simulink model "PreScan_Vissim_Python_0_cs_old"  (R2017b)
settings: Solver=ode5  StartTime=0.0  StopTime=inf  FixedStep=1/200  RelTol=1e-3
PreLoadFcn:
  | mbxruntime.callbacks.PreLoadFcn(bdroot);
PostLoadFcn:
  | mbxruntime.callbacks.PostLoadFcn(bdroot);
InitFcn:
  | mbxruntime.callbacks.InitFcn(bdroot);
StartFcn:
  | mbxruntime.callbacks.StartFcn(bdroot);
StopFcn:
  | mbxruntime.callbacks.StopFcn(bdroot);
model workspace (MAT data in the model file):
  mbox_table : struct (value not decoded)
  model_closed = 0
  sim_status = 0
undefined symbols (not defined in the file or in its folder): DiscIntNeverNeededParam
libraries: simulink x37, simulink_extras x12, PreScanSimulinkLibrary x11, dspnetwork x2, etargetslib x1, simulink_need_slupdate x1
(part 6 of 6)

== system PreScan_Vissim_Python_0_cs_old/Toyota_Yaris_Hatchback_1/Trajectories/Traj2State1/Traj2State2/Traj2MuxState_Ext/demux ==
  traj : Inport
  Demux : Demux  Outputs=18
  x : Outport
  y : Outport  Port=2
  z : Outport  Port=3
  velx : Outport  Port=4
  vely : Outport  Port=5
  velz : Outport  Port=6
  R : Outport  Port=7
  P : Outport  Port=8
  Y : Outport  Port=9
  velR : Outport  Port=10
  velP : Outport  Port=11
  velY : Outport  Port=12
  accx : Outport  Port=13
  accy : Outport  Port=14
  accz : Outport  Port=15
  accR : Outport  Port=16
  accP : Outport  Port=17
  accY : Outport  Port=18
  wires:
  Demux/18 -> accY/1
  Demux/17 -> accP/1
  Demux/16 -> accR/1
  Demux/15 -> accz/1
  Demux/14 -> accy/1
  Demux/13 -> accx/1
  Demux/12 -> velY/1
  Demux/11 -> velP/1
  Demux/10 -> velR/1
  Demux/9 -> velz/1
  Demux/8 -> vely/1
  Demux/7 -> velx/1
  Demux/6 -> Y/1
  Demux/5 -> P/1
  traj/1 -> Demux/1
  Demux/4 -> R/1
  Demux/3 -> z/1
  Demux/2 -> y/1
  Demux/1 -> x/1

== system PreScan_Vissim_Python_0_cs_old/Fiat_Bravo_Hatchback_1/Dynamics_Simple/Chassis/Bicycle_model_[XYZ]/X_Motion/Max RPM and zero- velocity detection/Configurable Subsystem ==
  Step : Step  Time=0.0001  Before=1  After=0  SampleTime=0
  Out1 : Outport
  wires:
  Step/1 -> Out1/1

== system PreScan_Vissim_Python_0_cs_old/Fiat_Bravo_Hatchback_1/Dynamics_Simple/Chassis/Bicycle_model_[XYZ]/X_Motion/Max RPM and zero- velocity detection/SR-Memory ==
  Signal : Inport
  Set : Inport  Port=2
  Reset : Inport  Port=3
  Constant : Constant  Value=0
  Detect Rise Positive : simulink/Logic and Bit Operations/Detect Rise Positive  vinit=0  InputProcessing=Inherited  OutDataTypeStr=uint8
  Detect Rise Positive1 : simulink/Logic and Bit Operations/Detect Rise Positive  vinit=0  InputProcessing=Inherited  OutDataTypeStr=uint8
  Manual Switch : ManualSwitch
  Manual Switch1 : ManualSwitch
  Switch : Switch  Criteria=u2 ~= 0
  Switch1 : Switch  Criteria=u2 ~= 0
  Unit Delay : UnitDelay  SampleTime=-1
  Out : Outport
  wires:
  Constant/1 -> Switch1/1
  Switch/1 -> Switch1/3
  Switch1/1 -> Unit Delay/1, Out/1
  Manual Switch1/1 -> Switch1/2
  Reset/1 -> Manual Switch1/2, Detect Rise Positive1/1
  Detect Rise Positive1/1 -> Manual Switch1/1
  Signal/1 -> Switch/1
  Unit Delay/1 -> Switch/3
  Set/1 -> Detect Rise Positive/1, Manual Switch/2
  Detect Rise Positive/1 -> Manual Switch/1
  Manual Switch/1 -> Switch/2

== system PreScan_Vissim_Python_0_cs_old/Toyota_Yaris_Hatchback_1/Dynamics_Simple/Chassis/Bicycle_model_[XYZ]/X_Motion/Max RPM and zero- velocity detection/Configurable Subsystem ==
  Step : Step  Time=0.0001  Before=1  After=0  SampleTime=0
  Out1 : Outport
  wires:
  Step/1 -> Out1/1

== system PreScan_Vissim_Python_0_cs_old/Toyota_Yaris_Hatchback_1/Dynamics_Simple/Chassis/Bicycle_model_[XYZ]/X_Motion/Max RPM and zero- velocity detection/SR-Memory ==
  Signal : Inport
  Set : Inport  Port=2
  Reset : Inport  Port=3
  Constant : Constant  Value=0
  Detect Rise Positive : simulink/Logic and Bit Operations/Detect Rise Positive  vinit=0  OutDataTypeStr=uint8
  Detect Rise Positive1 : simulink/Logic and Bit Operations/Detect Rise Positive  vinit=0  OutDataTypeStr=uint8
  Manual Switch : ManualSwitch
  Manual Switch1 : ManualSwitch
  Switch : Switch  Criteria=u2 ~= 0
  Switch1 : Switch  Criteria=u2 ~= 0
  Unit Delay : UnitDelay  SampleTime=-1
  Out : Outport
  wires:
  Constant/1 -> Switch1/1
  Switch/1 -> Switch1/3
  Switch1/1 -> Unit Delay/1, Out/1
  Manual Switch1/1 -> Switch1/2
  Reset/1 -> Manual Switch1/2, Detect Rise Positive1/1
  Detect Rise Positive1/1 -> Manual Switch1/1
  Signal/1 -> Switch/1
  Unit Delay/1 -> Switch/3
  Set/1 -> Detect Rise Positive/1, Manual Switch/2
  Detect Rise Positive/1 -> Manual Switch/1
  Manual Switch/1 -> Switch/2

== matlab function PreScan_Vissim_Python_0_cs_old/Toyota_Yaris_Hatchback_1/MATLAB Function6 ==
  data: u input; y1 output; y2 output; y3 output; y4 output; y5 output
function [y1,y2,y3,y4,y5]= fcn(u)

y1 = u(1);
y2 = u(2);
y3 = u(3);
y4 = u(4);
y5 = u(5);

== matlab function PreScan_Vissim_Python_0_cs_old/Toyota_Yaris_Hatchback_1/MATLAB Function1 ==
  data: x input; y output
function y = fcn(x)
y=0;
if (x>=750)
    y = 1;
end

== matlab function PreScan_Vissim_Python_0_cs_old/Toyota_Yaris_Hatchback_1/MATLAB Function ==
  data: u input; y output
function y = fcn(u)

y = u(1);
%pause(1);

== matlab function PreScan_Vissim_Python_0_cs_old/Toyota_Yaris_Hatchback_1/MATLAB Function7 ==
  data: IDs input; range input; azimuth input; send_data output; vel input; state input; if_collide input; Collid_1 input; Collid_2 input; if_road_end input
function send_data = fcn(IDs,range,azimuth ,vel ,state, if_collide,Collid_1,Collid_2,if_road_end)
coder.extrinsic('mat2str','disp','num2str','bdroot','get_param');


Number_data=10;
pt = 10;


t = num2str(round(get_param(bdroot,'SimulationTime'),pt),['%0' num2str(pt) '.2f ']);
% t = num2str(2.2,['%0.' num2str(pt) 'f ']);

To_add=['{"Time":"' t '", '];


for i=1:Number_data
    Id_name=num2str(i,['%0' num2str(3) '.f ']);
    Id_Colide=num2str(IDs(i),['%0' num2str(pt) '.f ']);
    Ra_Colide=num2str(range(i),['%0' num2str(pt) '.2f ']);
    az_Colide=num2str(azimuth(i),['%0' num2str(pt) '.2f ']);
    Ve_Colide=num2str(vel(i),['%0' num2str(pt) '.2f ']);
    
    
    To_add=[To_add '"Id' Id_name '":"' Id_Colide '", ' ...
                   '"Range' Id_name '":"' Ra_Colide '", ' ...
                   '"Azimuth' Id_name '":"' az_Colide '",' ...
                   '"Velocity' Id_name '":"' Ve_Colide '" '] ;
   if i<Number_data
       To_add=[To_add ', '];
   end
end

To_add=[To_add ', '];

pInput = 15;
pt = 10;
% % % % % % % % % % % % % % % % % 
p = pInput + 7;
state(isnan(state)) = 0;
u = zeros(9,p);
m = num2str([state(:);-1], ['% .' num2str(pInput) 'e ']);
sss = 1:p;
u(1,sss) = m(1,sss);    
u(2,sss) = m(2,sss);
u(3,sss) = m(3,sss);
u(4,sss) = m(4,sss);
u(5,sss) = m(5,sss);





To_add=[To_add '"Position":{"x":' u(1,:) ',"y":' u(2,:) '},' ...
        '"Velocity":' u(3,:) ',' ...
        '"Heading":' u(4,:) ',' ...
        '"Yaw":' u(5,:) ',' ];

% To_add=[To_add '"Position":{"x":' u(1,:) ',"y":' u(2,:) '},' ...
%         '"Velocity":' u(3,:) ',' ...
%         '"Heading":' u(3,:) ',' ...
%         '"Reward":' u(4,:) '}' ];
    
    
if_collide_s=num2str((if_collide),['%0' num2str(pt) '.f ']);
Collid_1_s=num2str(Collid_1,['%0' num2str(pt) '.f ']);
Collid_2_s=num2str(Collid_2,['%0' num2str(pt) '.f ']);

if_road_end_s=num2str((if_road_end),['%0' num2str(pt) '.f ']);


To_add=[To_add '"if_road_end":"' if_road_end_s '",'  ...
                '"if_collide":"' if_collide_s '",'  ...
                '"Collid_1":"' Collid_1_s '",'  ...
                '"Collid_2":"' Collid_2_s '"}'];


len=1306;
send_data = uint8(40*ones(len,1));

send_data = uint8(To_add);
send_data = uint8(send_data);

== matlab function PreScan_Vissim_Python_0_cs_old/Toyota_Yaris_Hatchback_1/PathFollower_1/CTRL REFERENCES/Find Reference Point (pref) on Trajectory closest to PVP Point (pvp)/eml_find_closest_trajectory_points ==
  data: pref output; Actor_traj_distance output; Actor_traj_angle output; pvp input; TrajOffset_x_y_Y input size=3; ActorOffset_Left_Right input; p0 input size=3; Traj_x parameter; Traj_y parameter
function [pref,Actor_traj_distance,Actor_traj_angle]  = eml_find_closest_trajectory_points(pvp,TrajOffset_x_y_Y,ActorOffset_Left_Right,p0,Traj_x,Traj_y)

[pref,Actor_traj_distance,Actor_traj_angle] = emlfcn_find_closest_trajectory_points(pvp,TrajOffset_x_y_Y,ActorOffset_Left_Right,p0,Traj_x,Traj_y,1);

end % end function

== matlab function PreScan_Vissim_Python_0_cs_old/Toyota_Yaris_Hatchback_1/PathFollower_1/DELTA CTRL/Calculate preview angle/eml_preview_angle_and_distance ==
  data: pvp input; alpha output; pref input; p0 input
function alpha = eml_preview_angle_and_distance(pvp, pref, p0)
%#eml

alpha = emlfcn_preview_angle_and_distance(pvp, pref, p0);

% end function
